simulink model "modelo"  (R2022b)
settings: Solver=ode45  StartTime=0.0  StopTime=100  RelTol=1e-3  EnableMultiTasking=on
values from neighbouring files (symbols this model uses):
  den = [50 43 3 1]    [control_experto.m]
  Kd = 0    [ZN.m]    (also in control_experto.m = Kp*Td; simular.m = pid(3))
  Ki = 0    [ZN.m]    (also in control_experto.m = Kp/Ti; simular.m = pid(2))
  Kp = 6*K    [control_experto.m]    (also in simular.m = pid(1))
  Mp = 100*(yp-ys)/ys    [caracteristicas.m]    (also in control_experto.m = input('  Sobreelongacion       : '); simular.m = 0)
  num = 1.5    [control_experto.m]
  tp = tout(ind(1))    [caracteristicas.m]    (also in control_experto.m = input('  Tiempo de pico        : '); simular.m = 0)
  tr = tout(ind(1))    [caracteristicas.m]    (also in control_experto.m = input('  Tiempo de subida      : '); simular.m = 0)
  ts = tout(i)    [caracteristicas.m]    (also in control_experto.m = input('  Tiempo de asentamiento: '); simular.m = 0)
  ys = yout(end)    [caracteristicas.m]    (also in control_experto.m = input('  Estado estacionario   : '); simular.m = 0)
libraries: simulink_need_slupdate x1
settings Model: Creator=heloi  LastModifiedBy=heloi
settings DataIOCC: SaveFormat=Array  SignalLoggingSaveFormat=ModelDataLogs  ReturnWorkspaceOutputs=off  SignalLoggingName=sigsOut
settings OptimizationCC: BooleanDataType=off
settings DebuggingCC: SaveWithParameterizedLinksMsg=none  UnderspecifiedInitializationDetection=Classic  MergeDetectMultiDrivingBlocksExec=none  SignalResolutionControl=TryResolveAllWithWarning  MultiTaskDSMMsg=warning  MultiTaskCondExecSysMsg=none  UnconnectedInputMsg=warning  UnconnectedOutputMsg=warning  UnconnectedLineMsg=warning
settings HardwareCC: ProdBitPerPointer=32  ProdBitPerSizeT=32  ProdBitPerPtrDiffT=32  ProdLargestAtomicFloat=None  ProdIntDivRoundTo=Undefined  ProdEndianess=Unspecified  ProdWordSize=32  ProdHWDeviceType=32-bit Generic  TargetUnknown=on
settings ModelReferenceCC: PropagateSignalLabelsOutOfModel=off
settings GRTTargetCC: CombineOutputUpdateFcns=off  GRTInterface=on
settings ConfigComp: CovMetricSettings=dw  CovSaveCumulativeToWorkspaceVar=on  CovSaveSingleToWorkspaceVar=on

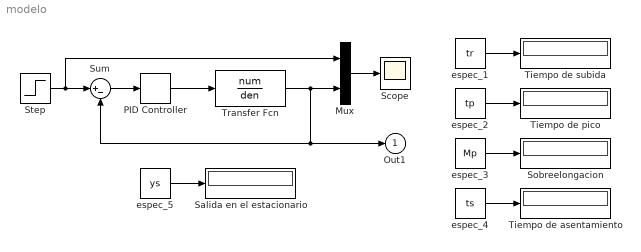
== system modelo ==
  Mux : Mux  Inputs=2
  PID Controller : simulink_need_slupdate/PID Controller  P=Kp + 0.5  I=Ki  D=Kd
  Salida en el estacionario : Display
  Scope : Scope
  Sobreelongacion : Display
  Step : Step  Time=0  SampleTime=0.01
  Sum : Sum  Inputs=|+-  InputSameDT=on  SaturateOnIntegerOverflow=on  OutDataTypeStr=Inherit: Same as first input
  Tiempo de asentamiento : Display
  Tiempo de pico : Display
  Tiempo de subida : Display
  Transfer Fcn : TransferFcn  Numerator=num  Denominator=den
  espec_1 : Constant  Value=tr
  espec_2 : Constant  Value=tp
  espec_3 : Constant  Value=Mp
  espec_4 : Constant  Value=ts
  espec_5 : Constant  Value=ys
  Out1 : Outport
  wires:
  Sum/1 -> PID Controller/1
  Step/1 -> Sum/1, Mux/1
  Mux/1 -> Scope/1
  PID Controller/1 -> Transfer Fcn/1
  Transfer Fcn/1 -> Mux/2, Sum/2, Out1/1
  espec_1/1 -> Tiempo de subida/1
  espec_2/1 -> Tiempo de pico/1
  espec_3/1 -> Sobreelongacion/1
  espec_4/1 -> Tiempo de asentamiento/1
  espec_5/1 -> Salida en el estacionario/1
